simulink model "Buck_DCM_Due"  (R2020a)
settings: Solver=FixedStepAuto  StartTime=0.0  StopTime=10  FixedStep=T  RelTol=1e-3  EnableMultiTasking=on
undefined symbols (not defined in the file): C, ILmax, Iumax, J, Ki_I, Ki_IL, Kp_I, Kp_IL, Kp_Uc, Kp_W, Kphi, L, Lu, rL, Ru, T, Ubat, Ucmax, wmax
libraries: arduinolib x20, simulink x16
(part 2 of 2)

== system Buck_DCM_Due/Speed Controller1 ==
  Mc : Inport
  w_mes : Inport  Port=2
  w_ref : Inport  Port=3
  P Controller : Gain  Gain=Kp_W
  Sum : Sum  Inputs=|++
  Sum1 : Sum  Inputs=|-+
  M_ref : Outport  InitialOutput=0  VectorParamsAs1DForOutWhenUnconnected=off
  wires:
  Sum/1 -> M_ref/1
  w_ref/1 -> Sum1/2
  Sum1/1 -> P Controller/1
  P Controller/1 -> Sum/2
  Mc/1 -> Sum/1
  w_mes/1 -> Sum1/1

== system Buck_DCM_Due/Speed Controller2 ==
  Mc : Inport
  w_mes : Inport  Port=2
  w_ref : Inport  Port=3
  P Controller : Gain  Gain=Kp_W
  Sum : Sum  Inputs=|++
  Sum1 : Sum  Inputs=|-+
  M_ref : Outport  InitialOutput=0  VectorParamsAs1DForOutWhenUnconnected=off
  wires:
  Sum/1 -> M_ref/1
  w_ref/1 -> Sum1/2
  Sum1/1 -> P Controller/1
  P Controller/1 -> Sum/2
  Mc/1 -> Sum/1
  w_mes/1 -> Sum1/1

== system Buck_DCM_Due/Uc Controller ==
  ILoad : Inport
  Uc_mes : Inport  Port=2
  Uc_ref : Inport  Port=3
  P Controller : Gain  Gain=Kp_Uc
  Saturation : Saturate  UpperLimit=ILmax  LowerLimit=0
  Sum : Sum  Inputs=++|
  Sum1 : Sum  Inputs=|-+
  IL_ref : Outport  InitialOutput=0
  wires:
  Uc_mes/1 -> Sum1/1
  Uc_ref/1 -> Sum1/2
  Sum1/1 -> P Controller/1
  P Controller/1 -> Sum/2
  ILoad/1 -> Sum/1
  Sum/1 -> Saturation/1
  Saturation/1 -> IL_ref/1

== system Buck_DCM_Due/Uc Controller1 ==
  ILoad : Inport
  Uc_mes : Inport  Port=2
  Uc_ref : Inport  Port=3
  P Controller : Gain  Gain=Kp_Uc
  Saturation : Saturate  UpperLimit=ILmax  LowerLimit=0
  Sum : Sum  Inputs=++|
  Sum1 : Sum  Inputs=|-+
  IL_ref : Outport  InitialOutput=0
  wires:
  Uc_mes/1 -> Sum1/1
  Uc_ref/1 -> Sum1/2
  Sum1/1 -> P Controller/1
  P Controller/1 -> Sum/2
  ILoad/1 -> Sum/1
  Sum/1 -> Saturation/1
  Saturation/1 -> IL_ref/1

== system Buck_DCM_Due/Uc Controller2 ==
  ILoad : Inport
  Uc_mes : Inport  Port=2
  Uc_ref : Inport  Port=3
  P Controller : Gain  Gain=Kp_Uc
  Saturation : Saturate  UpperLimit=ILmax  LowerLimit=0
  Sum : Sum  Inputs=++|
  Sum1 : Sum  Inputs=|-+
  IL_ref : Outport  InitialOutput=0
  wires:
  Uc_mes/1 -> Sum1/1
  Uc_ref/1 -> Sum1/2
  Sum1/1 -> P Controller/1
  P Controller/1 -> Sum/2
  ILoad/1 -> Sum/1
  Sum/1 -> Saturation/1
  Saturation/1 -> IL_ref/1
